simulink model "pll_digital"  (R2017b)
settings: Solver=ode1  StartTime=0.0  StopTime=0.2  FixedStep=1e-6  MaxStep=1e-4  RelTol=1e-3
InitFcn:
  | GlobalParam
undefined symbols (not defined in the file or in its folder): LL
libraries: powerlib x8, peTransforms x1, peSinusoidalMeasurement x1
settings Model: Creator=user  LastModifiedBy=user

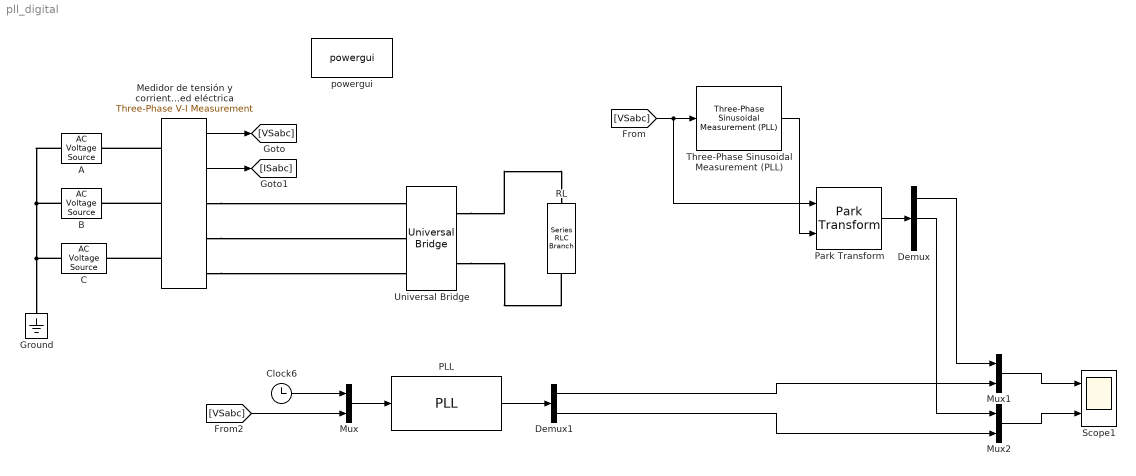
== system pll_digital ==
  "A " : powerlib/Electrical Sources/AC Voltage Source  Amplitude=1  Phase=0  Frequency=60  SampleTime=0  Measurements=None  BusType=swing  Pref=10e3  Qref=0  Qmin=-inf  Qmax=+inf
  "B " : powerlib/Electrical Sources/AC Voltage Source  Amplitude=1  Phase=-120  Frequency=60  SampleTime=0  Measurements=None  BusType=swing  Pref=10e3  Qref=0  Qmin=-inf  Qmax=+inf
  "C " : powerlib/Electrical Sources/AC Voltage Source  Amplitude=1  Phase=-240  Frequency=60  SampleTime=0  Measurements=None  BusType=swing  Pref=10e3  Qref=0  Qmin=-inf  Qmax=+inf
  Clock6 : Clock
  Demux : Demux  Outputs=3
  Demux1 : Demux  Outputs=2
  Ground : powerlib/Elements/Ground  LConnTagsString=a
  Medidor de tensión y corriente de la red eléctrica : powerlib/Measurements/Three-Phase V-I Measurement  VoltageMeasurement=phase-to-ground  SetLabelV=off  LabelV=Vabc  Vpu=off  VpuLL=off  CurrentMeasurement=yes  SetLabelI=off  LabelI=Iabc  Ipu=off  Pbase=100e6  Vbase=500e3  OutputType=Complex  PhasorSimulation=off  PSBequivalent=0
  Mux : Mux  Inputs=2
  Mux1 : Mux  Inputs=2
  Mux2 : Mux  Inputs=2
  "PLL " : MATLABFcn  MATLABFcn=PLL  OutputDimensions=2
  Park Transform : peTransforms/Park Transform  AxisAlignment=Q-axis  PowerInvariant=on
  "RL " : powerlib/Elements/Series RLC Branch  LConnTagsString=__new0  RConnTagsString=__new0  BranchType=R  Resistance=500  Inductance=LL  SetiL0=off  InitialCurrent=0  Capacitance=1e-6  Setx0=off  InitialVoltage=0  Measurements=None
  Scope1 : Scope  NumInputPorts=2
  Three-Phase Sinusoidal Measurement (PLL) : peSinusoidalMeasurement/Three-Phase Sinusoidal Measurement (PLL)  Kp_LF=222.1603  Ki_LF=25181.22  F0=60  Theta0=0  Ts=-1
  Universal Bridge : powerlib/Power Electronics/Universal Bridge  Arms=3  SnubberResistance=1e5  SnubberCapacitance=inf  Device=Diodes  Ron=1e-3  Lon=0  ForwardVoltages="[  0  0  ]"  ForwardVoltage=0  GTOparameters=[ 10e-6 , 20e-6 ]  IGBTparameters=[ 1e-6 , 2e-6 ]  Measurements=None  Measurements_2=None  converterType=Rectifier
  powergui : powerlib/powergui  Priority=1  SimulationMode=Discrete  SampleTime=5e-6  frequency=60  Iterations=50  frequencyindice=60  Pbase=100e6  ErrMax=1e-4  UnitsV=kV  UnitsW=MW  buscounter=0  FunctionMessages=off  echomessages=off  EnableUseOfTLC=off  CurrentSourceSwitches=off  DisableSnubberDevices=off  DisableRonSwitches=off  DisableVfSwitches=off  DisplayEquations=off  SolverType=Tustin/Backward Euler (TBE)  Interpol=off  ExternalGateDelay=off  methode=off  Ts=100  x0status=blocks  SPID=on  SwTol=0  HookPort=off  RestoreLinks=warning  ResistiveCurrentMeasurement=off  Frange=[0:2:500]  Ylog=off  Xlog=on  ShowGrid=off  save=off  variable=ZData  structure=0  ZoomFFT=off  StartTime=0.0  cycles=1  DisplayStyle=1  fundamental=60  FreqAxis=off  MaxFrequency=1000  frequencyindicesteady=1  RmsSteady=1  display=off
  wires:
  Medidor de tensión y corriente de la red eléctrica/1 -> [VSabc]
  Medidor de tensión y corriente de la red eléctrica/2 -> [ISabc]
  Mux/1 -> "PLL "/1
  Clock6/1 -> Mux/1
  [VSabc] -> Mux/2
  [VSabc] -> Park Transform/1, Three-Phase Sinusoidal Measurement (PLL)/1
  Three-Phase Sinusoidal Measurement (PLL)/2 -> Park Transform/2
  "PLL "/1 -> Demux1/1
  Park Transform/1 -> Demux/1
  Demux1/1 -> Mux1/2
  Mux1/1 -> Scope1/1
  Demux/1 -> Mux1/1
  Mux2/1 -> Scope1/2
  Demux1/2 -> Mux2/2
  Demux/2 -> Mux2/1
  connections:
  "B "/LConn1 -- "C "/LConn1 -- Ground/LConn1 -- "A "/LConn1
  Medidor de tensión y corriente de la red eléctrica/LConn2 -- "B "/RConn1
  Medidor de tensión y corriente de la red eléctrica/LConn1 -- "A "/RConn1
  Medidor de tensión y corriente de la red eléctrica/LConn3 -- "C "/RConn1
  Medidor de tensión y corriente de la red eléctrica/RConn1 -- Universal Bridge/LConn1
  Medidor de tensión y corriente de la red eléctrica/RConn3 -- Universal Bridge/LConn3
  Medidor de tensión y corriente de la red eléctrica/RConn2 -- Universal Bridge/LConn2
  Universal Bridge/RConn2 -- "RL "/RConn1
  Universal Bridge/RConn1 -- "RL "/LConn1
